simulink model "Pricing_Harvey_Delay_Attack"  (R2020b)
settings: Solver=ode5  StartTime=0.0  StopTime=1  FixedStep=0.001  RelTol=1e-3
settings Model: Creator=SEAL_Admin  LastModifiedBy=SEAL_Admin
settings DataIOCC: SaveOutput=off  SaveTime=off
settings OptimizationCC: BlockReduction=off  OptimizeBlockIOStorage=off

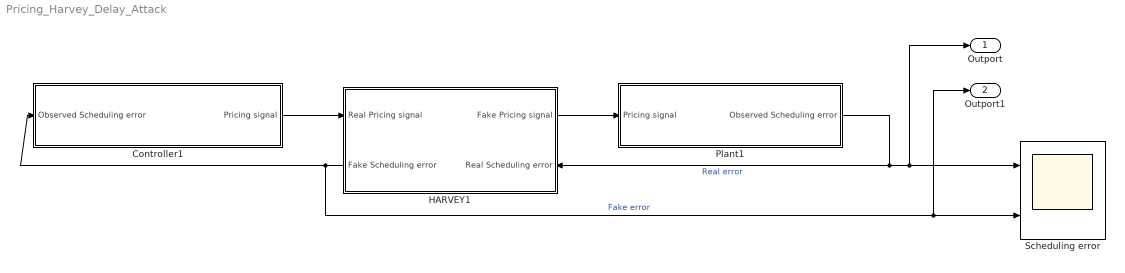
== system Pricing_Harvey_Delay_Attack ==
  Controller1 : Subsystem
  HARVEY1 : Subsystem
      settings: PortSchema="{\"entries\":[{\"content\":{\"sides\":[{\"content\":{\"connectorIds\":[\"In1\",\"Out2\"]},\"type\":\"ConnectorPlacement.EquallySpacedRectSide\",\"uuid\":\"a539da20-d974-4e5f-b08d-2d7e07e26864\"},{\"content\":{\"connectorIds\":[\"Out1\",\"In2\"],\"side\":\"RIGHT\"},\"type\":\"ConnectorPlacement.EquallySpacedRectSide\",\"uuid\":\"9eef7b98-1a08-4c57-94a1-c2fb8561f6b7\"},{\"content\":{\"connectorIds\":[],\"side\":\"TOP\"},\"type\":\"ConnectorPlacement.EquallySpacedRectSide\",\"uuid\":\"bcefc905-0f7f-4ff9-9e92-375db830387e\"},{\"content\":{\"connectorIds\":[],\"side\":\"HIDDEN\"},\"type\":\"ConnectorPlacement.EquallySpacedRectSide\",\"uuid\":\"852d0f69-157a-4ba1-a6ae-e0df46c0c703\"}]},\"type\":\"ConnectorPlacement.EquallySpacedConnector\",\"uuid\":\"59eab357-4454-48ca-9daf-4caa40877b03\"}],\"packageUris\":[\"http://schema.mathworks.com/mf0/Connector/R2020b\"],\"version\":\"1.0\"}"
  Plant1 : Subsystem
  Scheduling error : Scope  NumInputPorts=2
  Outport : Outport
  Outport1 : Outport  Port=2
  wires:
  HARVEY1/1(Fake Pricing signal) -> Plant1/1(Pricing signal)
  Plant1/1(Observed Scheduling error) -> HARVEY1/2(Real Scheduling error), Outport/1, Scheduling error/1  "Real error"
  HARVEY1/2(Fake Scheduling error) -> Outport1/1, Scheduling error/2, Controller1/1(Observed Scheduling error)  "Fake error"
  Controller1/1(Pricing signal) -> HARVEY1/1(Real Pricing signal)

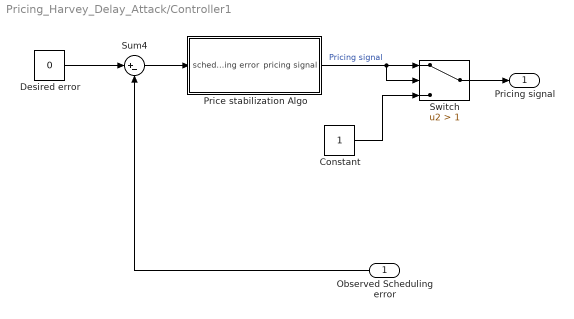
== system Pricing_Harvey_Delay_Attack/Controller1 ==
  Observed Scheduling error : Inport
  Constant : Constant
  Desired error : Constant  Value=0
  Price stabilization Algo : Subsystem
  Sum4 : Sum  Inputs=|+-
  Switch : Switch  Criteria=u2 > Threshold  Threshold=1
  Pricing signal : Outport
  wires:
  Sum4/1 -> Price stabilization Algo/1(scheduling error)
  Desired error/1 -> Sum4/1
  Price stabilization Algo/1(pricing signal) -> Switch/2, Switch/1  "Pricing signal"
  Observed Scheduling error/1 -> Sum4/2
  Switch/1 -> Pricing signal/1
  Constant/1 -> Switch/3

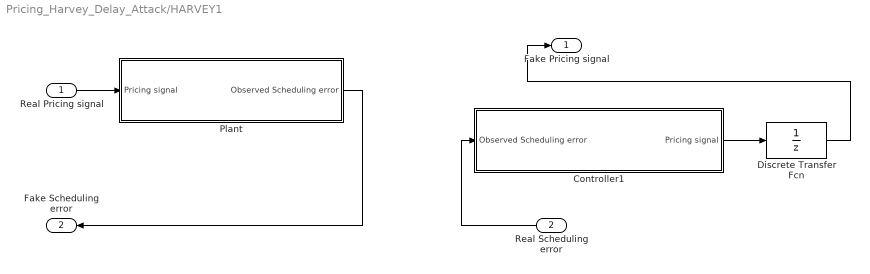
== system Pricing_Harvey_Delay_Attack/HARVEY1 ==
  Real Pricing signal : Inport
  Real Scheduling error : Inport  Port=2
  Controller1 : Subsystem
  Discrete Transfer Fcn : DiscreteTransferFcn  Denominator=[1 0]
  Plant : Subsystem
  Fake Pricing signal : Outport
  Fake Scheduling error : Outport  Port=2
  wires:
  Real Pricing signal/1 -> Plant/1(Pricing signal)
  Plant/1(Observed Scheduling error) -> Fake Scheduling error/1
  Real Scheduling error/1 -> Controller1/1(Observed Scheduling error)
  Controller1/1(Pricing signal) -> Discrete Transfer Fcn/1
  Discrete Transfer Fcn/1 -> Fake Pricing signal/1

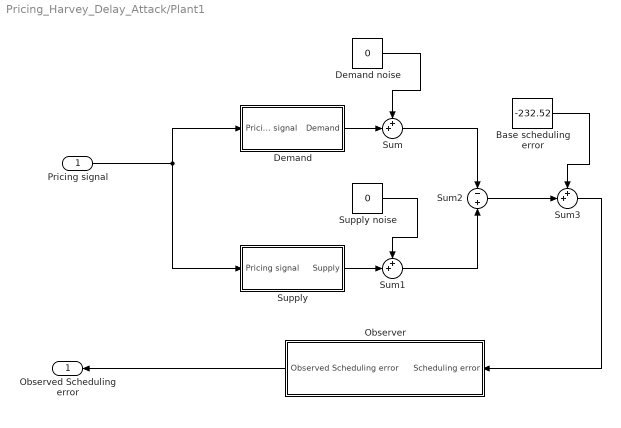
== system Pricing_Harvey_Delay_Attack/Plant1 ==
  Pricing signal : Inport
  Base scheduling error : Constant  Value=-232.52
  Demand : Subsystem
  Demand noise : Constant  Value=0
  Observer : Subsystem
  Sum : Sum  Inputs=++|
  Sum1 : Sum  Inputs=++|
  Sum2 : Sum  Inputs=-|+
  Sum3 : Sum  Inputs=++|
  Supply : Subsystem
  Supply noise : Constant  Value=0
  Observed Scheduling error : Outport
  wires:
  Sum1/1 -> Sum2/2
  Sum3/1 -> Observer/1(Scheduling error)
  Sum2/1 -> Sum3/2
  Supply noise/1 -> Sum1/1
  Supply/1(Supply) -> Sum1/2
  Pricing signal/1 -> Supply/1(Pricing signal), Demand/1(Pricing signal)
  Demand noise/1 -> Sum/1
  Sum/1 -> Sum2/1
  Demand/1(Demand) -> Sum/2
  Base scheduling error/1 -> Sum3/1
  Observer/1(Observed Scheduling error) -> Observed Scheduling error/1

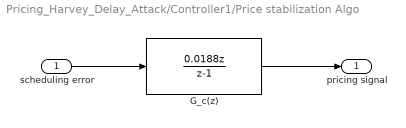
== system Pricing_Harvey_Delay_Attack/Controller1/Price stabilization Algo ==
  scheduling error : Inport
  G_c(z) : DiscreteTransferFcn  Numerator=[0.0188 0]  Denominator=[1 -1]
  pricing signal : Outport
  wires:
  scheduling error/1 -> G_c(z)/1
  G_c(z)/1 -> pricing signal/1

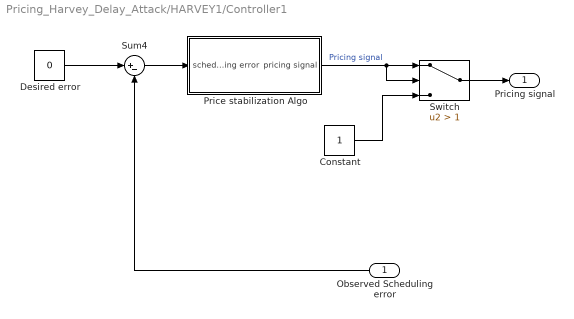
== system Pricing_Harvey_Delay_Attack/HARVEY1/Controller1 ==
  Observed Scheduling error : Inport
  Constant : Constant
  Desired error : Constant  Value=0
  Price stabilization Algo : Subsystem
  Sum4 : Sum  Inputs=|+-
  Switch : Switch  Criteria=u2 > Threshold  Threshold=1
  Pricing signal : Outport
  wires:
  Sum4/1 -> Price stabilization Algo/1(scheduling error)
  Desired error/1 -> Sum4/1
  Price stabilization Algo/1(pricing signal) -> Switch/2, Switch/1  "Pricing signal"
  Observed Scheduling error/1 -> Sum4/2
  Switch/1 -> Pricing signal/1
  Constant/1 -> Switch/3

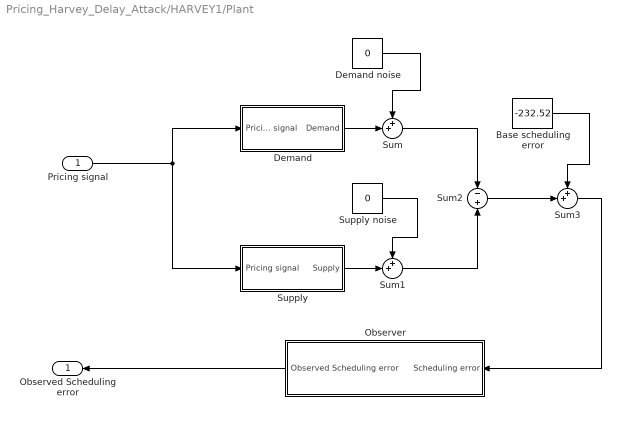
== system Pricing_Harvey_Delay_Attack/HARVEY1/Plant ==
  Pricing signal : Inport
  Base scheduling error : Constant  Value=-232.52
  Demand : Subsystem
  Demand noise : Constant  Value=0
  Observer : Subsystem
  Sum : Sum  Inputs=++|
  Sum1 : Sum  Inputs=++|
  Sum2 : Sum  Inputs=-|+
  Sum3 : Sum  Inputs=++|
  Supply : Subsystem
  Supply noise : Constant  Value=0
  Observed Scheduling error : Outport
  wires:
  Sum1/1 -> Sum2/2
  Sum3/1 -> Observer/1(Scheduling error)
  Sum2/1 -> Sum3/2
  Supply noise/1 -> Sum1/1
  Supply/1(Supply) -> Sum1/2
  Pricing signal/1 -> Supply/1(Pricing signal), Demand/1(Pricing signal)
  Demand noise/1 -> Sum/1
  Sum/1 -> Sum2/1
  Demand/1(Demand) -> Sum/2
  Base scheduling error/1 -> Sum3/1
  Observer/1(Observed Scheduling error) -> Observed Scheduling error/1

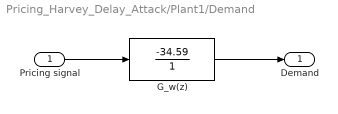
== system Pricing_Harvey_Delay_Attack/Plant1/Demand ==
  Pricing signal : Inport
  G_w(z) : TransferFcn  Numerator=[-34.59]  Denominator=[0 1]
  Demand : Outport
  wires:
  Pricing signal/1 -> G_w(z)/1
  G_w(z)/1 -> Demand/1

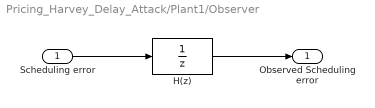
== system Pricing_Harvey_Delay_Attack/Plant1/Observer ==
  Scheduling error : Inport
  H(z) : DiscreteTransferFcn  Denominator=[1 0]
  Observed Scheduling error : Outport
  wires:
  Scheduling error/1 -> H(z)/1
  H(z)/1 -> Observed Scheduling error/1

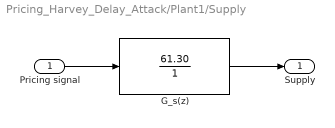
== system Pricing_Harvey_Delay_Attack/Plant1/Supply ==
  Pricing signal : Inport
  G_s(z) : TransferFcn  Numerator=[61.30]  Denominator=[0 1]
  Supply : Outport
  wires:
  Pricing signal/1 -> G_s(z)/1
  G_s(z)/1 -> Supply/1

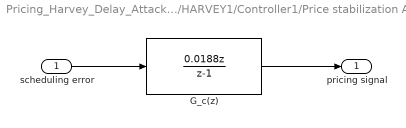
== system Pricing_Harvey_Delay_Attack/HARVEY1/Controller1/Price stabilization Algo ==
  scheduling error : Inport
  G_c(z) : DiscreteTransferFcn  Numerator=[0.0188 0]  Denominator=[1 -1]
  pricing signal : Outport
  wires:
  scheduling error/1 -> G_c(z)/1
  G_c(z)/1 -> pricing signal/1

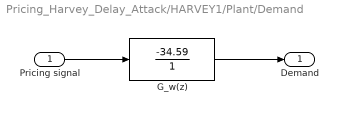
== system Pricing_Harvey_Delay_Attack/HARVEY1/Plant/Demand ==
  Pricing signal : Inport
  G_w(z) : TransferFcn  Numerator=[-34.59]  Denominator=[0 1]
  Demand : Outport
  wires:
  Pricing signal/1 -> G_w(z)/1
  G_w(z)/1 -> Demand/1

== system Pricing_Harvey_Delay_Attack/HARVEY1/Plant/Observer ==
  Scheduling error : Inport
  H(z) : DiscreteTransferFcn  Denominator=[1 0]
  Observed Scheduling error : Outport
  wires:
  Scheduling error/1 -> H(z)/1
  H(z)/1 -> Observed Scheduling error/1

== system Pricing_Harvey_Delay_Attack/HARVEY1/Plant/Supply ==
  Pricing signal : Inport
  G_s(z) : TransferFcn  Numerator=[61.30]  Denominator=[0 1]
  Supply : Outport
  wires:
  Pricing signal/1 -> G_s(z)/1
  G_s(z)/1 -> Supply/1
